simulink model "Hysteresis"  (R2020a)
settings: Solver=FixedStepAuto  StartTime=0.0  StopTime=10.0  FixedStep=1e-3  RelTol=1e-3  EnableMultiTasking=on
settings Model: ExtModeTrigDuration=5  Creator=liams  LastModifiedBy=liams
settings OptimizationCC: EnhancedBackFolding=on  PassReuseOutputArgsAs=Individual arguments  ZeroExternalMemoryAtStartup=off  ZeroInternalMemoryAtStartup=off  MaxStackSize=64  OptimizeBlockOrder=speed  DifferentSizesBufferReuse=on  OptimizationCustomize=off  EfficientTunableParamExpr=on
settings DebuggingCC: ParameterTunabilityLossMsg=error
settings HardwareCC: ProdBitPerPointer=32  ProdBitPerSizeT=32  ProdBitPerPtrDiffT=32  ProdLargestAtomicInteger=Long  ProdLargestAtomicFloat=Double  ProdWordSize=32  ProdHWDeviceType=ARM Compatible->ARM Cortex
settings SFSimCC: MATLABDynamicMemAlloc=off
settings RTWCC: SystemTargetFile=ert.tlc  HardwareBoard=NXP FRDM-K64F  TemplateMakefile=ert_default_tmf  Toolchain=GNU Tools for ARM Embedded Processors
settings CodeAppCC: ForceParamTrailComments=on  IgnoreCustomStorageClasses=off  OperatorAnnotations=on  SimulinkDataObjDesc=on  SFDataObjDesc=on  InsertBlockDesc=on

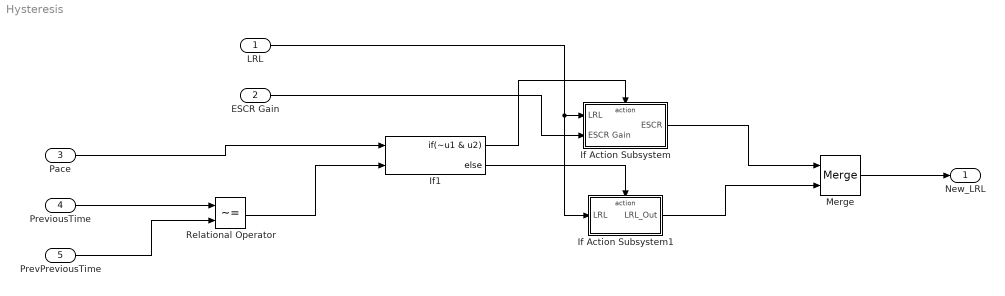
== system Hysteresis ==
  LRL : Inport
  ESCR Gain : Inport  Port=2
  Pace : Inport  Port=3  OutDataTypeStr=boolean
  PreviousTime : Inport  Port=4
  PrevPreviousTime : Inport  Port=5
  If Action Subsystem : Subsystem  TreatAsAtomicUnit=on
  If Action Subsystem1 : Subsystem  TreatAsAtomicUnit=on
  If1 : If  NumInputs=2  IfExpression=~u1 & u2
  Merge : Merge
  Relational Operator : RelationalOperator  Operator=~=  OutDataTypeStr=boolean  RndMeth=Simplest
  New_LRL : Outport
  wires:
  If Action Subsystem/1(ESCR) -> Merge/1
  If Action Subsystem1/1(LRL_Out) -> Merge/2
  Merge/1 -> New_LRL/1
  PreviousTime/1 -> Relational Operator/1
  PrevPreviousTime/1 -> Relational Operator/2
  Pace/1 -> If1/1
  Relational Operator/1 -> If1/2
  If1/1 -> If Action Subsystem/Action
  If1/2 -> If Action Subsystem1/Action
  LRL/1 -> If Action Subsystem1/1(LRL), If Action Subsystem/1(LRL)
  ESCR Gain/1 -> If Action Subsystem/2(ESCR Gain)

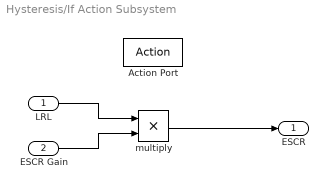
== system Hysteresis/If Action Subsystem ==
  LRL : Inport
  ESCR Gain : Inport  Port=2
  Action Port : ActionPort  ActionPortLabel=if(~u1 & u2)
  multiply : Product  Inputs=**
  ESCR : Outport
  wires:
  LRL/1 -> multiply/1
  ESCR Gain/1 -> multiply/2
  multiply/1 -> ESCR/1

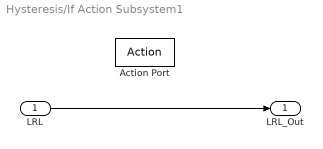
== system Hysteresis/If Action Subsystem1 ==
  LRL : Inport
  Action Port : ActionPort  ActionPortLabel=else
  LRL_Out : Outport
  wires:
  LRL/1 -> LRL_Out/1
